simulink model "MiniDroneLogicalArchitecture"  (R2022a)
settings: Solver=VariableStepAuto  StartTime=0.0  StopTime=10.0  RelTol=1e-3
settings Model: DataDictionary=MiniDroneArchData.sldd  Creator=tshifera  LastModifiedBy=tobia

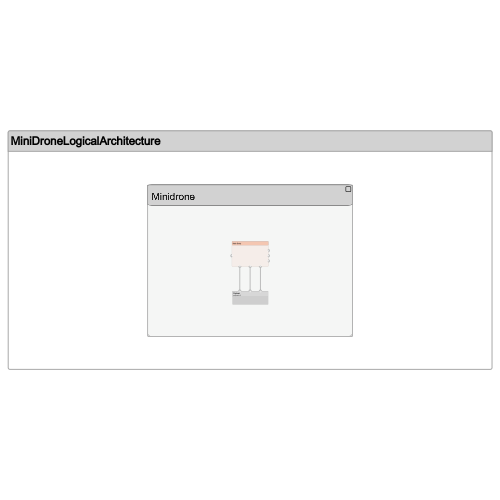
[thumbnail: Simulink's stored preview of the top-level diagram]
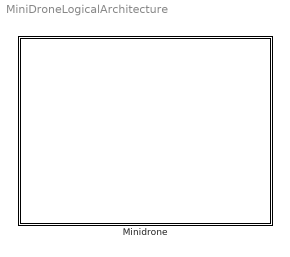
== system MiniDroneLogicalArchitecture ==
  Minidrone : Subsystem
      settings: PortSchema="{\"entries\":[{\"content\":{\"headerSize\":26,\"margin\":15,\"minimumSpacing\":25,\"sides\":[{\"content\":{\"connectorIds\":[]},\"type\":\"ConnectorPlacement.EquallySpacedRectSide\",\"uuid\":\"58971a95-43ec-4e42-90cb-f52848a43a78\"},{\"content\":{\"connectorIds\":[],\"side\":\"RIGHT\"},\"type\":\"ConnectorPlacement.EquallySpacedRectSide\",\"uuid\":\"43bd139b-3ebd-443e-9d04-2758c166e5e5\"},{\"content\":{\"connectorIds\":[],\"side\":\"TOP\"},\"type\":\"ConnectorPlacement.EquallySpacedRectSide\",\"uuid\":\"9440dd5a-d47a-4e7e-9dec-7137884490cd\"}]},\"type\":\"ConnectorPlacement.EquallySpacedConnector\",\"uuid\":\"fbcd83c6-9a27-4688-9f1d-1a4d28d86620\"}],\"packageUris\":[\"http://schema.mathworks.com/mf0/Connector/R2020b\"],\"version\":\"1.0\"}"

== system MiniDroneLogicalArchitecture/Minidrone ==
  Main Vehicle : Subsystem
      settings: PortSchema="{\"entries\":[{\"content\":{\"headerSize\":26,\"margin\":15,\"minimumSpacing\":25,\"sides\":[{\"content\":{\"connectorIds\":[\"In2\"]},\"type\":\"ConnectorPlacement.EquallySpacedRectSide\",\"uuid\":\"58971a95-43ec-4e42-90cb-f52848a43a78\"},{\"content\":{\"connectorIds\":[\"Out1\",\"Out2\",\"Out5\"],\"side\":\"RIGHT\"},\"type\":\"ConnectorPlacement.EquallySpacedRectSide\",\"uuid\":\"43bd139b-3ebd-443e-9d04-2758c166e5e5\"},{\"content\":{\"connectorIds\":[],\"side\":\"TOP\"},\"type\":\"ConnectorPlacement.EquallySpacedRectSide\",\"uuid\":\"9440dd5a-d47a-4e7e-9dec-7137884490cd\"},{\"content\":{\"connectorIds\":[\"Out3\",\"Out4\",\"In1\"],\"side\":\"BOTTOM\"},\"type\":\"ConnectorPlacement.EquallySpacedRectSide\",\"uuid\":\"027f250f-1c99-4780-b31a-0472dacd58c4\"}]},\"type\":\"ConnectorPlacement.EquallySpacedConnector\",\"uuid\":\"fbcd83c6-9a27-4688-9f1d-1a4d28d86620\"}],\"packageUris\":[\"http://schema.mathworks.com/mf0/Connector/R2020b\"],\"version\":\"1.0\"}"
  Payload : Subsystem  Variant=on
      settings: PortSchema="{\"entries\":[{\"content\":{\"headerSize\":38,\"margin\":15,\"minimumSpacing\":25,\"sides\":[{\"content\":{\"connectorIds\":[]},\"type\":\"ConnectorPlacement.EquallySpacedRectSide\",\"uuid\":\"bb20ca61-cc69-46ba-bbf8-c616735728e4\"},{\"content\":{\"connectorIds\":[],\"side\":\"RIGHT\"},\"type\":\"ConnectorPlacement.EquallySpacedRectSide\",\"uuid\":\"ae599026-5f79-458c-a34f-615f09cd605e\"},{\"content\":{\"connectorIds\":[\"In1\",\"In2\",\"Out1\"],\"side\":\"TOP\"},\"type\":\"ConnectorPlacement.EquallySpacedRectSide\",\"uuid\":\"37784589-cb93-414b-b17d-4791bb265658\"}]},\"type\":\"ConnectorPlacement.EquallySpacedConnector\",\"uuid\":\"a9e16083-13fe-49b9-9fa3-3eed0fc58f12\"}],\"packageUris\":[\"http://schema.mathworks.com/mf0/Connector/R2020b\"],\"version\":\"1.0\"}"
  wires:
  Main Vehicle/3(PL Coupling) -> Payload/1(PL Coupling)
  Main Vehicle/4(PL Command) -> Payload/2(PL Command)
  Payload/1(PL State) -> Main Vehicle/1(PL State)

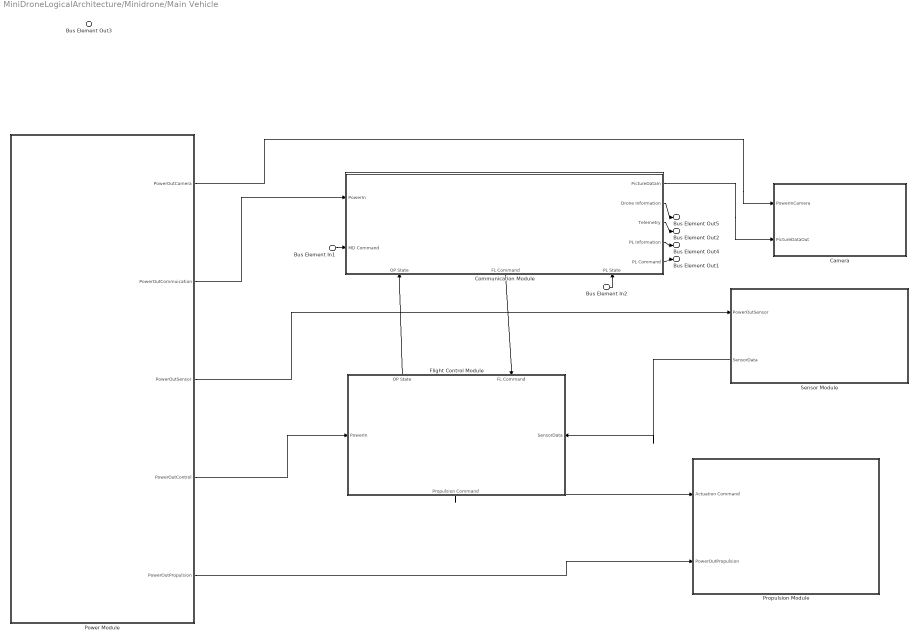
== system MiniDroneLogicalArchitecture/Minidrone/Main Vehicle ==
  Bus Element In2 : Inport  PortName=PL State
  Bus Element In1 : Inport  Port=2  PortName=MD Command
  Camera : Subsystem  VariantControl=payload==1
      settings: PortSchema="{\"entries\":[{\"content\":{\"headerSize\":26,\"margin\":15,\"minimumSpacing\":25,\"sides\":[{\"content\":{\"connectorIds\":[\"In1\",\"In2\"]},\"type\":\"ConnectorPlacement.EquallySpacedRectSide\",\"uuid\":\"62dbea54-6b04-428b-9082-afe16aec4c16\"},{\"content\":{\"connectorIds\":[],\"side\":\"RIGHT\"},\"type\":\"ConnectorPlacement.EquallySpacedRectSide\",\"uuid\":\"bd8afa16-d094-436c-bc9f-80902768e85a\"},{\"content\":{\"connectorIds\":[],\"side\":\"TOP\"},\"type\":\"ConnectorPlacement.EquallySpacedRectSide\",\"uuid\":\"5bc22b2d-7b46-48f6-9c81-aea78f4cffe8\"}]},\"type\":\"ConnectorPlacement.EquallySpacedConnector\",\"uuid\":\"869dc23c-b8e9-4489-a84c-3bf9ddec322d\"}],\"packageUris\":[\"http://schema.mathworks.com/mf0/Connector/R2020b\"],\"version\":\"1.0\"}"
  Communication Module : Subsystem
      settings: PortSchema="{\"entries\":[{\"content\":{\"headerSize\":26,\"margin\":15,\"minimumSpacing\":25,\"sides\":[{\"content\":{\"connectorIds\":[\"In3\",\"In4\"]},\"type\":\"ConnectorPlacement.EquallySpacedRectSide\",\"uuid\":\"11745183-c785-42ff-bcc1-ca3285cfe892\"},{\"content\":{\"connectorIds\":[\"Out1\",\"Out2\",\"Out6\",\"Out4\",\"Out5\"],\"side\":\"RIGHT\"},\"type\":\"ConnectorPlacement.EquallySpacedRectSide\",\"uuid\":\"762d8cad-319e-4e1e-8739-8b76a70aa4c0\"},{\"content\":{\"connectorIds\":[],\"side\":\"TOP\"},\"type\":\"ConnectorPlacement.EquallySpacedRectSide\",\"uuid\":\"cf327f13-56fb-47e7-82e2-9b80047871fd\"},{\"content\":{\"connectorIds\":[\"In1\",\"Out3\",\"In2\"],\"side\":\"BOTTOM\"},\"type\":\"ConnectorPlacement.EquallySpacedRectSide\",\"uuid\":\"b154881a-f2db-4811-b63b-30ed04e21acf\"}]},\"type\":\"ConnectorPlacement.EquallySpacedConnector\",\"uuid\":\"6e856333-11ed-42a7-b683-e6a750f8e1be\"}],\"packageUris\":[\"http://schema.mathworks.com/mf0/Connector/R2020b\"],\"version\":\"1.0\"}"
  Flight Control Module : Subsystem
      settings: PortSchema="{\"entries\":[{\"content\":{\"headerSize\":26,\"margin\":15,\"minimumSpacing\":25,\"sides\":[{\"content\":{\"connectorIds\":[\"In2\"]},\"type\":\"ConnectorPlacement.EquallySpacedRectSide\",\"uuid\":\"11745183-c785-42ff-bcc1-ca3285cfe892\"},{\"content\":{\"connectorIds\":[\"In3\"],\"side\":\"RIGHT\"},\"type\":\"ConnectorPlacement.EquallySpacedRectSide\",\"uuid\":\"762d8cad-319e-4e1e-8739-8b76a70aa4c0\"},{\"content\":{\"connectorIds\":[\"Out1\",\"In1\"],\"side\":\"TOP\"},\"type\":\"ConnectorPlacement.EquallySpacedRectSide\",\"uuid\":\"cf327f13-56fb-47e7-82e2-9b80047871fd\"},{\"content\":{\"connectorIds\":[\"Out2\"],\"side\":\"BOTTOM\"},\"type\":\"ConnectorPlacement.EquallySpacedRectSide\",\"uuid\":\"d4b2c298-dd23-4e2a-8fa6-8732704f5c39\"}]},\"type\":\"ConnectorPlacement.EquallySpacedConnector\",\"uuid\":\"6e856333-11ed-42a7-b683-e6a750f8e1be\"}],\"packageUris\":[\"http://schema.mathworks.com/mf0/Connector/R2020b\"],\"version\":\"1.0\"}"
  Power Module : Subsystem
      settings: PortSchema="{\"entries\":[{\"content\":{\"headerSize\":26,\"margin\":15,\"minimumSpacing\":25,\"sides\":[{\"content\":{\"connectorIds\":[]},\"type\":\"ConnectorPlacement.EquallySpacedRectSide\",\"uuid\":\"11745183-c785-42ff-bcc1-ca3285cfe892\"},{\"content\":{\"connectorIds\":[\"Out1\",\"Out5\",\"Out3\",\"Out2\",\"Out4\"],\"side\":\"RIGHT\"},\"type\":\"ConnectorPlacement.EquallySpacedRectSide\",\"uuid\":\"762d8cad-319e-4e1e-8739-8b76a70aa4c0\"},{\"content\":{\"connectorIds\":[],\"side\":\"TOP\"},\"type\":\"ConnectorPlacement.EquallySpacedRectSide\",\"uuid\":\"cf327f13-56fb-47e7-82e2-9b80047871fd\"}]},\"type\":\"ConnectorPlacement.EquallySpacedConnector\",\"uuid\":\"6e856333-11ed-42a7-b683-e6a750f8e1be\"}],\"packageUris\":[\"http://schema.mathworks.com/mf0/Connector/R2020b\"],\"version\":\"1.0\"}"
  Propulsion Module : Subsystem
      settings: PortSchema="{\"entries\":[{\"content\":{\"headerSize\":26,\"margin\":15,\"minimumSpacing\":25,\"sides\":[{\"content\":{\"connectorIds\":[\"In1\",\"In2\"]},\"type\":\"ConnectorPlacement.EquallySpacedRectSide\",\"uuid\":\"11745183-c785-42ff-bcc1-ca3285cfe892\"},{\"content\":{\"connectorIds\":[],\"side\":\"RIGHT\"},\"type\":\"ConnectorPlacement.EquallySpacedRectSide\",\"uuid\":\"762d8cad-319e-4e1e-8739-8b76a70aa4c0\"},{\"content\":{\"connectorIds\":[],\"side\":\"TOP\"},\"type\":\"ConnectorPlacement.EquallySpacedRectSide\",\"uuid\":\"cf327f13-56fb-47e7-82e2-9b80047871fd\"}]},\"type\":\"ConnectorPlacement.EquallySpacedConnector\",\"uuid\":\"6e856333-11ed-42a7-b683-e6a750f8e1be\"}],\"packageUris\":[\"http://schema.mathworks.com/mf0/Connector/R2020b\"],\"version\":\"1.0\"}"
  Sensor Module : Subsystem
      settings: PortSchema="{\"entries\":[{\"content\":{\"headerSize\":26,\"margin\":15,\"minimumSpacing\":25,\"sides\":[{\"content\":{\"connectorIds\":[\"In1\",\"Out1\"]},\"type\":\"ConnectorPlacement.EquallySpacedRectSide\",\"uuid\":\"11745183-c785-42ff-bcc1-ca3285cfe892\"},{\"content\":{\"connectorIds\":[],\"side\":\"RIGHT\"},\"type\":\"ConnectorPlacement.EquallySpacedRectSide\",\"uuid\":\"762d8cad-319e-4e1e-8739-8b76a70aa4c0\"},{\"content\":{\"connectorIds\":[],\"side\":\"TOP\"},\"type\":\"ConnectorPlacement.EquallySpacedRectSide\",\"uuid\":\"cf327f13-56fb-47e7-82e2-9b80047871fd\"}]},\"type\":\"ConnectorPlacement.EquallySpacedConnector\",\"uuid\":\"6e856333-11ed-42a7-b683-e6a750f8e1be\"}],\"packageUris\":[\"http://schema.mathworks.com/mf0/Connector/R2020b\"],\"version\":\"1.0\"}"
  Bus Element Out5 : Outport  PortName=Drone Information
  Bus Element Out4 : Outport  Port=2  PortName=PL Information
  Bus Element Out3 : Outport  Port=3  PortName=PL Coupling
  Bus Element Out1 : Outport  Port=4  PortName=PL Command
  Bus Element Out2 : Outport  Port=5  PortName=Telemetry
  wires:
  Bus Element In1/1 -> Communication Module/4(MD Command)
  Communication Module/3(FL Command) -> Flight Control Module/1(FL Command)
  Power Module/5(PowerOutCommuication) -> Communication Module/3(PowerIn)
  Power Module/2(PowerOutControl) -> Flight Control Module/2(PowerIn)
  Power Module/4(PowerOutPropulsion) -> Propulsion Module/2(PowerOutPropulsion)
  Communication Module/6(Telemetry) -> Bus Element Out2/1
  Flight Control Module/1(OP State) -> Communication Module/1(OP State)
  Communication Module/5(PL Command) -> Bus Element Out1/1
  Bus Element In2/1 -> Communication Module/2(PL State)
  Communication Module/4(PL Information) -> Bus Element Out4/1
  Communication Module/2(Drone Information) -> Bus Element Out5/1
  Sensor Module/1(SensorData) -> Flight Control Module/3(SensorData)
  Flight Control Module/2(Propulsion Command) -> Propulsion Module/1(Actuation Command)
  Power Module/3(PowerOutSensor) -> Sensor Module/1(PowerOutSensor)
  Power Module/1(PowerOutCamera) -> Camera/1(PowerInCamera)
  Communication Module/1(PictureDataIn) -> Camera/2(PictureDataOut)

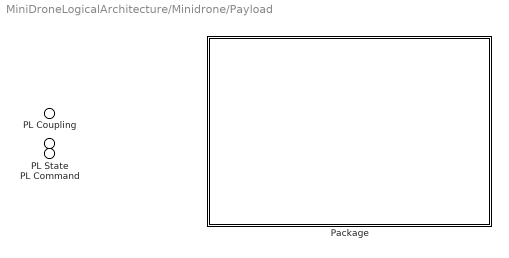
== system MiniDroneLogicalArchitecture/Minidrone/Payload ==
  PL Coupling : Inport
  PL Command : Inport  Port=2
  Package : Subsystem  VariantControl=payload==2
      settings: PortSchema="{\"entries\":[{\"content\":{\"headerSize\":26,\"margin\":15,\"minimumSpacing\":25,\"sides\":[{\"content\":{\"connectorIds\":[]},\"type\":\"ConnectorPlacement.EquallySpacedRectSide\",\"uuid\":\"62dbea54-6b04-428b-9082-afe16aec4c16\"},{\"content\":{\"connectorIds\":[],\"side\":\"RIGHT\"},\"type\":\"ConnectorPlacement.EquallySpacedRectSide\",\"uuid\":\"bd8afa16-d094-436c-bc9f-80902768e85a\"},{\"content\":{\"connectorIds\":[],\"side\":\"TOP\"},\"type\":\"ConnectorPlacement.EquallySpacedRectSide\",\"uuid\":\"5bc22b2d-7b46-48f6-9c81-aea78f4cffe8\"}]},\"type\":\"ConnectorPlacement.EquallySpacedConnector\",\"uuid\":\"869dc23c-b8e9-4489-a84c-3bf9ddec322d\"}],\"packageUris\":[\"http://schema.mathworks.com/mf0/Connector/R2020b\"],\"version\":\"1.0\"}"
  PL State : Outport

== system MiniDroneLogicalArchitecture/Minidrone/Main Vehicle/Camera ==
  Bus Element In1 : Inport  PortName=PowerInCamera
  Bus Element In2 : Inport  Port=2  PortName=PictureDataOut

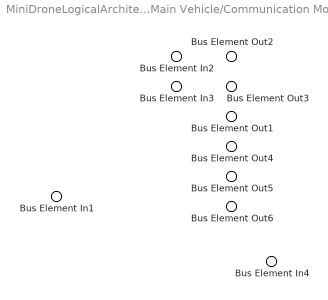
== system MiniDroneLogicalArchitecture/Minidrone/Main Vehicle/Communication Module ==
  Bus Element In4 : Inport  PortName=OP State
  Bus Element In3 : Inport  Port=2  PortName=PL State
  Bus Element In2 : Inport  Port=3  PortName=PowerIn
  Bus Element In1 : Inport  Port=4  PortName=MD Command
  Bus Element Out6 : Outport  PortName=PictureDataIn
  Bus Element Out5 : Outport  Port=2  PortName=Drone Information
  Bus Element Out2 : Outport  Port=3  PortName=FL Command
  Bus Element Out4 : Outport  Port=4  PortName=PL Information
  Bus Element Out1 : Outport  Port=5  PortName=PL Command
  Bus Element Out3 : Outport  Port=6  PortName=Telemetry

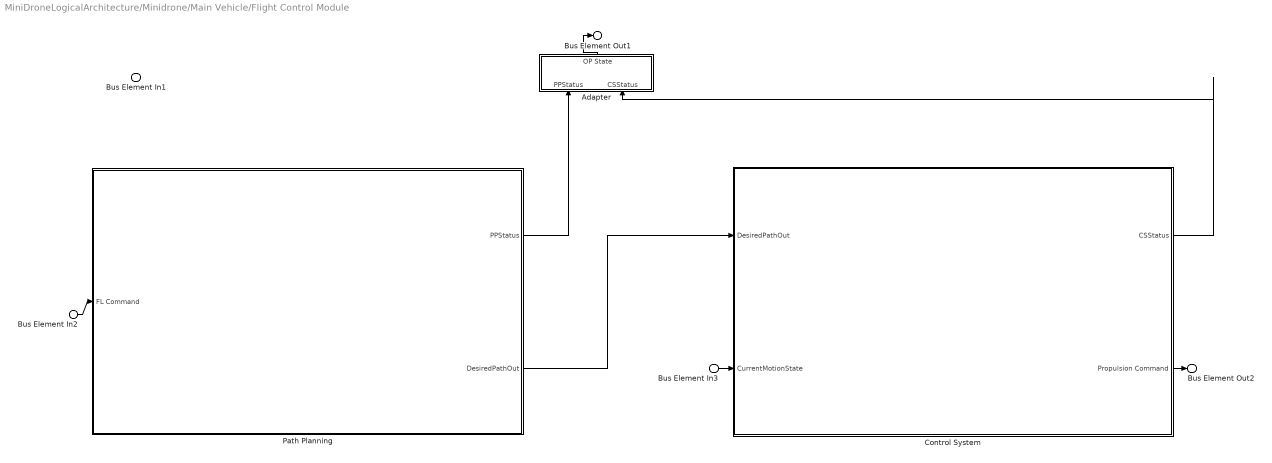
== system MiniDroneLogicalArchitecture/Minidrone/Main Vehicle/Flight Control Module ==
  Bus Element In2 : Inport  PortName=FL Command
  Bus Element In1 : Inport  Port=2  PortName=PowerIn
  Bus Element In3 : Inport  Port=3  PortName=SensorData
  Adapter : Subsystem
      settings: PortSchema="{\"entries\":[{\"content\":{\"margin\":10,\"minimumSpacing\":15,\"sides\":[{\"content\":{\"connectorIds\":[]},\"type\":\"ConnectorPlacement.EquallySpacedRectSide\",\"uuid\":\"8029eac4-1e93-42cb-93bf-2741aac18114\"},{\"content\":{\"connectorIds\":[],\"side\":\"RIGHT\"},\"type\":\"ConnectorPlacement.EquallySpacedRectSide\",\"uuid\":\"880550d5-d396-4c9d-9596-cf9ff815056e\"},{\"content\":{\"connectorIds\":[\"Out1\"],\"side\":\"TOP\"},\"type\":\"ConnectorPlacement.EquallySpacedRectSide\",\"uuid\":\"ddd57148-5a11-4830-bb53-0e7c5eb0188d\"},{\"content\":{\"connectorIds\":[\"In1\",\"In2\"],\"side\":\"BOTTOM\"},\"type\":\"ConnectorPlacement.EquallySpacedRectSide\",\"uuid\":\"686e057f-801d-4689-adbf-8d23a9ad6c3b\"}]},\"type\":\"ConnectorPlacement.EquallySpacedConnector\",\"uuid\":\"9cd7aed1-ed17-433b-a42b-f5bc10fbd0dd\"}],\"packageUris\":[\"http://schema.mathworks.com/mf0/Connector/R2020b\"],\"version\":\"1.0\"}"
  Control System : Subsystem
      settings: PortSchema="{\"entries\":[{\"content\":{\"headerSize\":26,\"margin\":15,\"minimumSpacing\":25,\"sides\":[{\"content\":{\"connectorIds\":[\"In1\",\"In2\"]},\"type\":\"ConnectorPlacement.EquallySpacedRectSide\",\"uuid\":\"11745183-c785-42ff-bcc1-ca3285cfe892\"},{\"content\":{\"connectorIds\":[\"Out1\",\"Out2\"],\"side\":\"RIGHT\"},\"type\":\"ConnectorPlacement.EquallySpacedRectSide\",\"uuid\":\"762d8cad-319e-4e1e-8739-8b76a70aa4c0\"},{\"content\":{\"connectorIds\":[],\"side\":\"TOP\"},\"type\":\"ConnectorPlacement.EquallySpacedRectSide\",\"uuid\":\"cf327f13-56fb-47e7-82e2-9b80047871fd\"}]},\"type\":\"ConnectorPlacement.EquallySpacedConnector\",\"uuid\":\"6e856333-11ed-42a7-b683-e6a750f8e1be\"}],\"packageUris\":[\"http://schema.mathworks.com/mf0/Connector/R2020b\"],\"version\":\"1.0\"}"
  Path Planning : Subsystem
      settings: PortSchema="{\"entries\":[{\"content\":{\"headerSize\":26,\"margin\":15,\"minimumSpacing\":25,\"sides\":[{\"content\":{\"connectorIds\":[\"In1\"]},\"type\":\"ConnectorPlacement.EquallySpacedRectSide\",\"uuid\":\"11745183-c785-42ff-bcc1-ca3285cfe892\"},{\"content\":{\"connectorIds\":[\"Out1\",\"Out2\"],\"side\":\"RIGHT\"},\"type\":\"ConnectorPlacement.EquallySpacedRectSide\",\"uuid\":\"762d8cad-319e-4e1e-8739-8b76a70aa4c0\"},{\"content\":{\"connectorIds\":[],\"side\":\"TOP\"},\"type\":\"ConnectorPlacement.EquallySpacedRectSide\",\"uuid\":\"cf327f13-56fb-47e7-82e2-9b80047871fd\"}]},\"type\":\"ConnectorPlacement.EquallySpacedConnector\",\"uuid\":\"6e856333-11ed-42a7-b683-e6a750f8e1be\"}],\"packageUris\":[\"http://schema.mathworks.com/mf0/Connector/R2020b\"],\"version\":\"1.0\"}"
  Bus Element Out1 : Outport  PortName=OP State
  Bus Element Out2 : Outport  Port=2  PortName=Propulsion Command
  wires:
  Bus Element In2/1 -> Path Planning/1(FL Command)
  Path Planning/2(DesiredPathOut) -> Control System/1(DesiredPathOut)
  Bus Element In3/1 -> Control System/2(CurrentMotionState)
  Control System/2(Propulsion Command) -> Bus Element Out2/1
  Adapter/1(OP State) -> Bus Element Out1/1
  Path Planning/1(PPStatus) -> Adapter/1(PPStatus)
  Control System/1(CSStatus) -> Adapter/2(CSStatus)

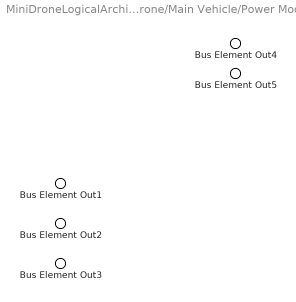
== system MiniDroneLogicalArchitecture/Minidrone/Main Vehicle/Power Module ==
  Bus Element Out5 : Outport  PortName=PowerOutCamera
  Bus Element Out1 : Outport  Port=2  PortName=PowerOutControl
  Bus Element Out4 : Outport  Port=3  PortName=PowerOutSensor
  Bus Element Out2 : Outport  Port=4  PortName=PowerOutPropulsion
  Bus Element Out3 : Outport  Port=5  PortName=PowerOutCommuication

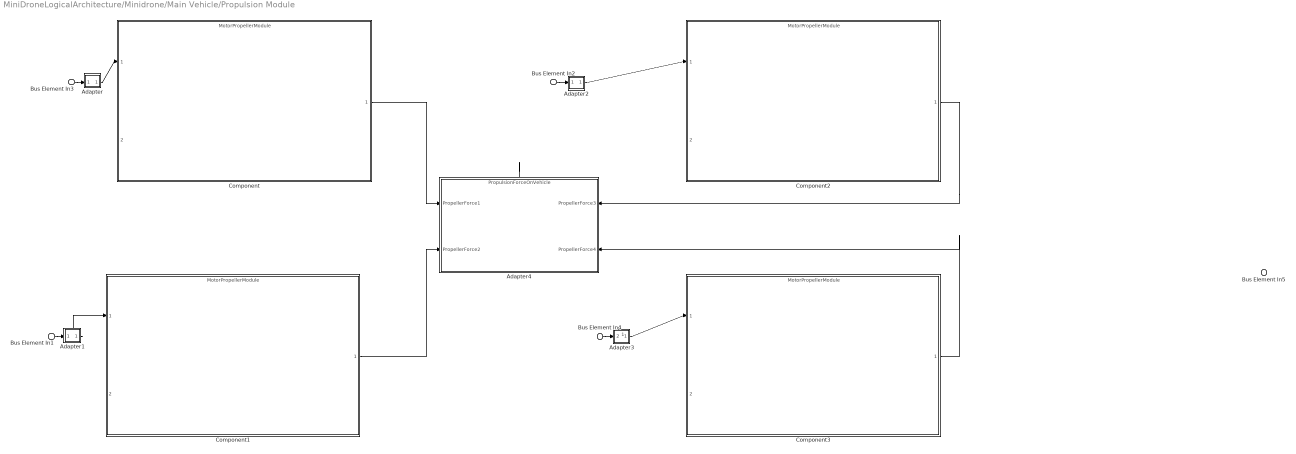
== system MiniDroneLogicalArchitecture/Minidrone/Main Vehicle/Propulsion Module ==
  Bus Element In{1..4} (4 alike) : Inport  PortName=Actuation Command
  Bus Element In5 : Inport  Port=2  PortName=PowerOutPropulsion
  Adapter : Subsystem
      settings: PortSchema="{\"entries\":[{\"content\":{\"margin\":10,\"minimumSpacing\":15,\"sides\":[{\"content\":{\"connectorIds\":[\"In1\"]},\"type\":\"ConnectorPlacement.EquallySpacedRectSide\",\"uuid\":\"8029eac4-1e93-42cb-93bf-2741aac18114\"},{\"content\":{\"connectorIds\":[\"Out1\"],\"side\":\"RIGHT\"},\"type\":\"ConnectorPlacement.EquallySpacedRectSide\",\"uuid\":\"880550d5-d396-4c9d-9596-cf9ff815056e\"},{\"content\":{\"connectorIds\":[],\"side\":\"TOP\"},\"type\":\"ConnectorPlacement.EquallySpacedRectSide\",\"uuid\":\"ddd57148-5a11-4830-bb53-0e7c5eb0188d\"}]},\"type\":\"ConnectorPlacement.EquallySpacedConnector\",\"uuid\":\"9cd7aed1-ed17-433b-a42b-f5bc10fbd0dd\"}],\"packageUris\":[\"http://schema.mathworks.com/mf0/Connector/R2020b\"],\"version\":\"1.0\"}"
  Adapter1 : Subsystem
      settings: PortSchema="{\"entries\":[{\"content\":{\"margin\":10,\"minimumSpacing\":15,\"sides\":[{\"content\":{\"connectorIds\":[\"In1\"]},\"type\":\"ConnectorPlacement.EquallySpacedRectSide\",\"uuid\":\"8029eac4-1e93-42cb-93bf-2741aac18114\"},{\"content\":{\"connectorIds\":[\"Out1\"],\"side\":\"RIGHT\"},\"type\":\"ConnectorPlacement.EquallySpacedRectSide\",\"uuid\":\"880550d5-d396-4c9d-9596-cf9ff815056e\"},{\"content\":{\"connectorIds\":[],\"side\":\"TOP\"},\"type\":\"ConnectorPlacement.EquallySpacedRectSide\",\"uuid\":\"ddd57148-5a11-4830-bb53-0e7c5eb0188d\"}]},\"type\":\"ConnectorPlacement.EquallySpacedConnector\",\"uuid\":\"9cd7aed1-ed17-433b-a42b-f5bc10fbd0dd\"}],\"packageUris\":[\"http://schema.mathworks.com/mf0/Connector/R2020b\"],\"version\":\"1.0\"}"
  Adapter2 : Subsystem
      settings: PortSchema="{\"entries\":[{\"content\":{\"margin\":10,\"minimumSpacing\":15,\"sides\":[{\"content\":{\"connectorIds\":[\"In1\"]},\"type\":\"ConnectorPlacement.EquallySpacedRectSide\",\"uuid\":\"8029eac4-1e93-42cb-93bf-2741aac18114\"},{\"content\":{\"connectorIds\":[\"Out1\"],\"side\":\"RIGHT\"},\"type\":\"ConnectorPlacement.EquallySpacedRectSide\",\"uuid\":\"880550d5-d396-4c9d-9596-cf9ff815056e\"},{\"content\":{\"connectorIds\":[],\"side\":\"TOP\"},\"type\":\"ConnectorPlacement.EquallySpacedRectSide\",\"uuid\":\"ddd57148-5a11-4830-bb53-0e7c5eb0188d\"}]},\"type\":\"ConnectorPlacement.EquallySpacedConnector\",\"uuid\":\"9cd7aed1-ed17-433b-a42b-f5bc10fbd0dd\"}],\"packageUris\":[\"http://schema.mathworks.com/mf0/Connector/R2020b\"],\"version\":\"1.0\"}"
  Adapter3 : Subsystem
      settings: PortSchema="{\"entries\":[{\"content\":{\"margin\":10,\"minimumSpacing\":15,\"sides\":[{\"content\":{\"connectorIds\":[\"In2\"]},\"type\":\"ConnectorPlacement.EquallySpacedRectSide\",\"uuid\":\"8029eac4-1e93-42cb-93bf-2741aac18114\"},{\"content\":{\"connectorIds\":[\"Out1\"],\"side\":\"RIGHT\"},\"type\":\"ConnectorPlacement.EquallySpacedRectSide\",\"uuid\":\"880550d5-d396-4c9d-9596-cf9ff815056e\"},{\"content\":{\"connectorIds\":[\"In1\"],\"side\":\"TOP\"},\"type\":\"ConnectorPlacement.EquallySpacedRectSide\",\"uuid\":\"ddd57148-5a11-4830-bb53-0e7c5eb0188d\"}]},\"type\":\"ConnectorPlacement.EquallySpacedConnector\",\"uuid\":\"9cd7aed1-ed17-433b-a42b-f5bc10fbd0dd\"}],\"packageUris\":[\"http://schema.mathworks.com/mf0/Connector/R2020b\"],\"version\":\"1.0\"}"
  Adapter4 : Subsystem
      settings: PortSchema="{\"entries\":[{\"content\":{\"margin\":10,\"minimumSpacing\":15,\"sides\":[{\"content\":{\"connectorIds\":[\"In4\",\"In3\"]},\"type\":\"ConnectorPlacement.EquallySpacedRectSide\",\"uuid\":\"b95fdf5c-7c32-4cea-a1d5-46e14885b6c7\"},{\"content\":{\"connectorIds\":[\"In1\",\"In2\"],\"side\":\"RIGHT\"},\"type\":\"ConnectorPlacement.EquallySpacedRectSide\",\"uuid\":\"406c0812-4108-47cf-89cd-ae4270ca37a8\"},{\"content\":{\"connectorIds\":[\"Out1\"],\"side\":\"TOP\"},\"type\":\"ConnectorPlacement.EquallySpacedRectSide\",\"uuid\":\"1ebf6b83-00c0-4ac6-93de-25d0ef6ef9e5\"}]},\"type\":\"ConnectorPlacement.EquallySpacedConnector\",\"uuid\":\"7218703e-d378-431b-88e9-2d6710b1e02c\"}],\"packageUris\":[\"http://schema.mathworks.com/mf0/Connector/R2020b\"],\"version\":\"1.0\"}"
  Component{,1..3} (4 alike) : ModelReference  ModelNameDialog=MotorPropellerModule.slx  SimulationMode=Normal  ModelReferenceVersion=1.7
      settings: PortSchema="{\"entries\":[{\"content\":{\"headerSize\":38,\"margin\":15,\"minimumSpacing\":25,\"sides\":[{\"content\":{\"connectorIds\":[\"In1\",\"In2\"]},\"type\":\"ConnectorPlacement.EquallySpacedRectSide\",\"uuid\":\"7b7af72e-aa04-46fd-a07e-d8d59d662379\"},{\"content\":{\"connectorIds\":[\"Out1\"],\"side\":\"RIGHT\"},\"type\":\"ConnectorPlacement.EquallySpacedRectSide\",\"uuid\":\"fdfbdd79-f6fe-4609-8655-22f9d8d17dc0\"},{\"content\":{\"connectorIds\":[],\"side\":\"TOP\"},\"type\":\"ConnectorPlacement.EquallySpacedRectSide\",\"uuid\":\"626fe178-dafd-47c5-aa64-f4cd4b451539\"}]},\"type\":\"ConnectorPlacement.EquallySpacedConnector\",\"uuid\":\"b35cf388-f6ba-41d8-a395-5e8a060747f6\"}],\"packageUris\":[\"http://schema.mathworks.com/mf0/Connector/R2020b\"],\"version\":\"1.0\"}"
  wires:
  Adapter/1(MotorCommand) -> Component/1
  Bus Element In3/1 -> Adapter/1(Actuation Command)
  Adapter1/1(MotorCommand) -> Component1/1
  Bus Element In1/1 -> Adapter1/1(Actuation Command)
  Adapter2/1(MotorCommand) -> Component2/1
  Bus Element In2/1 -> Adapter2/1(Actuation Command)
  Bus Element In4/1 -> Adapter3/2(Actuation Command)
  Adapter3/1(MotorCommand) -> Component3/1
  Adapter4/1(PropulsionForceOnVehicle) -> ?
  Component2/1 -> Adapter4/1(PropellerForce3)
  Component3/1 -> Adapter4/2(PropellerForce4)
  Component1/1 -> Adapter4/3(PropellerForce2)
  Component/1 -> Adapter4/4(PropellerForce1)

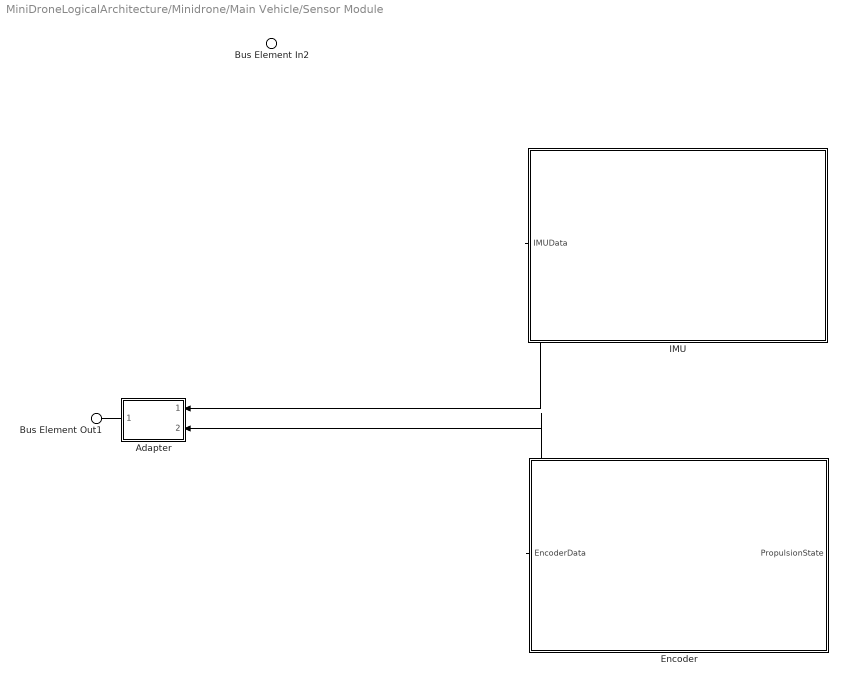
== system MiniDroneLogicalArchitecture/Minidrone/Main Vehicle/Sensor Module ==
  Bus Element In2 : Inport  PortName=PowerOutSensor
  Adapter : Subsystem
      settings: PortSchema="{\"entries\":[{\"content\":{\"margin\":10,\"minimumSpacing\":15,\"sides\":[{\"content\":{\"connectorIds\":[\"Out1\"]},\"type\":\"ConnectorPlacement.EquallySpacedRectSide\",\"uuid\":\"58971a95-43ec-4e42-90cb-f52848a43a78\"},{\"content\":{\"connectorIds\":[\"In1\",\"In2\"],\"side\":\"RIGHT\"},\"type\":\"ConnectorPlacement.EquallySpacedRectSide\",\"uuid\":\"43bd139b-3ebd-443e-9d04-2758c166e5e5\"},{\"content\":{\"connectorIds\":[],\"side\":\"TOP\"},\"type\":\"ConnectorPlacement.EquallySpacedRectSide\",\"uuid\":\"9440dd5a-d47a-4e7e-9dec-7137884490cd\"},{\"content\":{\"connectorIds\":[],\"side\":\"BOTTOM\"},\"type\":\"ConnectorPlacement.EquallySpacedRectSide\",\"uuid\":\"a500e90f-9d10-4320-8532-1d80de54d601\"}]},\"type\":\"ConnectorPlacement.EquallySpacedConnector\",\"uuid\":\"fbcd83c6-9a27-4688-9f1d-1a4d28d86620\"}],\"packageUris\":[\"http://schema.mathworks.com/mf0/Connector/R2020b\"],\"version\":\"1.0\"}"
  Encoder : Subsystem
      settings: PortSchema="{\"entries\":[{\"content\":{\"headerSize\":26,\"margin\":15,\"minimumSpacing\":25,\"sides\":[{\"content\":{\"connectorIds\":[\"Out1\"]},\"type\":\"ConnectorPlacement.EquallySpacedRectSide\",\"uuid\":\"58971a95-43ec-4e42-90cb-f52848a43a78\"},{\"content\":{\"connectorIds\":[\"In1\"],\"side\":\"RIGHT\"},\"type\":\"ConnectorPlacement.EquallySpacedRectSide\",\"uuid\":\"43bd139b-3ebd-443e-9d04-2758c166e5e5\"},{\"content\":{\"connectorIds\":[],\"side\":\"TOP\"},\"type\":\"ConnectorPlacement.EquallySpacedRectSide\",\"uuid\":\"9440dd5a-d47a-4e7e-9dec-7137884490cd\"}]},\"type\":\"ConnectorPlacement.EquallySpacedConnector\",\"uuid\":\"fbcd83c6-9a27-4688-9f1d-1a4d28d86620\"}],\"packageUris\":[\"http://schema.mathworks.com/mf0/Connector/R2020b\"],\"version\":\"1.0\"}"
  "IMU " : Subsystem
      settings: PortSchema="{\"entries\":[{\"content\":{\"headerSize\":26,\"margin\":15,\"minimumSpacing\":25,\"sides\":[{\"content\":{\"connectorIds\":[\"Out1\"]},\"type\":\"ConnectorPlacement.EquallySpacedRectSide\",\"uuid\":\"58971a95-43ec-4e42-90cb-f52848a43a78\"},{\"content\":{\"connectorIds\":[],\"side\":\"RIGHT\"},\"type\":\"ConnectorPlacement.EquallySpacedRectSide\",\"uuid\":\"43bd139b-3ebd-443e-9d04-2758c166e5e5\"},{\"content\":{\"connectorIds\":[],\"side\":\"TOP\"},\"type\":\"ConnectorPlacement.EquallySpacedRectSide\",\"uuid\":\"9440dd5a-d47a-4e7e-9dec-7137884490cd\"}]},\"type\":\"ConnectorPlacement.EquallySpacedConnector\",\"uuid\":\"fbcd83c6-9a27-4688-9f1d-1a4d28d86620\"}],\"packageUris\":[\"http://schema.mathworks.com/mf0/Connector/R2020b\"],\"version\":\"1.0\"}"
  Bus Element Out1 : Outport  PortName=SensorData
  wires:
  ? -> Encoder/1(PropulsionState)
  Adapter/1(SensorData) -> Bus Element Out1/1
  "IMU "/1(IMUData) -> Adapter/1(IMUData)
  Encoder/1(EncoderData) -> Adapter/2(EncoderData)

== system MiniDroneLogicalArchitecture/Minidrone/Payload/Package ==

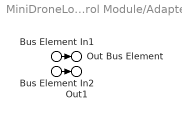
== system MiniDroneLogicalArchitecture/Minidrone/Main Vehicle/Flight Control Module/Adapter ==
  Bus Element In1 : Inport  PortName=PPStatus
  Bus Element In2 : Inport  Port=2  PortName=CSStatus
  Out Bus Element : Outport  PortName=OP State  Element=PPStatus
  Out1 : Outport  PortName=OP State  Element=CSStatus
  wires:
  Bus Element In1/1 -> Out Bus Element/1
  Bus Element In2/1 -> Out1/1

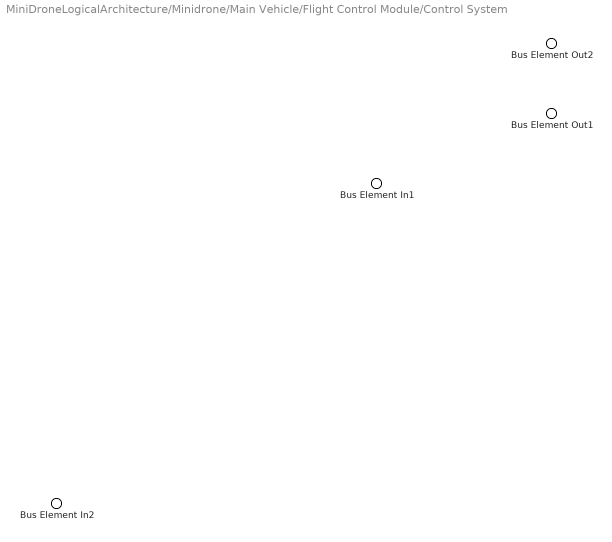
== system MiniDroneLogicalArchitecture/Minidrone/Main Vehicle/Flight Control Module/Control System ==
  Bus Element In1 : Inport  PortName=DesiredPathOut
  Bus Element In2 : Inport  Port=2  PortName=CurrentMotionState
  Bus Element Out2 : Outport  PortName=CSStatus
  Bus Element Out1 : Outport  Port=2  PortName=Propulsion Command

== system MiniDroneLogicalArchitecture/Minidrone/Main Vehicle/Flight Control Module/Path Planning ==
  Bus Element In1 : Inport  PortName=FL Command
  Bus Element Out2 : Outport  PortName=PPStatus
  Bus Element Out1 : Outport  Port=2  PortName=DesiredPathOut

== system MiniDroneLogicalArchitecture/Minidrone/Main Vehicle/Propulsion Module/Adapter ==
  In Bus Element : Inport  PortName=Actuation Command  Element=elem0
  Out Bus Element : Outport  PortName=MotorCommand
  wires:
  In Bus Element/1 -> Out Bus Element/1

== system MiniDroneLogicalArchitecture/Minidrone/Main Vehicle/Propulsion Module/Adapter1 ==
  In Bus Element : Inport  PortName=Actuation Command  Element=elem1
  Out Bus Element : Outport  PortName=MotorCommand
  wires:
  In Bus Element/1 -> Out Bus Element/1

== system MiniDroneLogicalArchitecture/Minidrone/Main Vehicle/Propulsion Module/Adapter2 ==
  In Bus Element : Inport  PortName=Actuation Command  Element=elem2
  Out Bus Element : Outport  PortName=MotorCommand
  wires:
  In Bus Element/1 -> Out Bus Element/1

== system MiniDroneLogicalArchitecture/Minidrone/Main Vehicle/Propulsion Module/Adapter3 ==
  Bus Element In1 : Inport  PortName=InBus
  In Bus Element : Inport  Port=2  PortName=Actuation Command  Element=elem3
  Out Bus Element : Outport  PortName=MotorCommand
  wires:
  In Bus Element/1 -> Out Bus Element/1

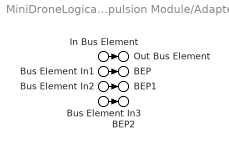
== system MiniDroneLogicalArchitecture/Minidrone/Main Vehicle/Propulsion Module/Adapter4 ==
  Bus Element In2 : Inport  PortName=PropellerForce3
  Bus Element In3 : Inport  Port=2  PortName=PropellerForce4
  Bus Element In1 : Inport  Port=3  PortName=PropellerForce2
  In Bus Element : Inport  Port=4  PortName=PropellerForce1
  Out Bus Element : Outport  PortName=PropulsionForceOnVehicle  Element=ForcePropeller1
  BEP : Outport  PortName=PropulsionForceOnVehicle  Element=ForcePropeller2
  BEP1 : Outport  PortName=PropulsionForceOnVehicle  Element=ForcePropeller3
  BEP2 : Outport  PortName=PropulsionForceOnVehicle  Element=ForcePropeller4
  wires:
  In Bus Element/1 -> Out Bus Element/1
  Bus Element In1/1 -> BEP/1
  Bus Element In2/1 -> BEP1/1
  Bus Element In3/1 -> BEP2/1

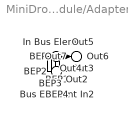
== system MiniDroneLogicalArchitecture/Minidrone/Main Vehicle/Sensor Module/Adapter ==
  In Bus Element : Inport  PortName=IMUData  Element=Acceleration
  BEP : Inport  PortName=IMUData  Element=AngularAcceleration
  BEP1 : Inport  PortName=IMUData  Element=Pose
  Bus Element In2 : Inport  Port=2  PortName=EncoderData  Element=Motor1Velocity
  BEP2 : Inport  Port=2  PortName=EncoderData  Element=Motor2Velocity
  BEP3 : Inport  Port=2  PortName=EncoderData  Element=Motor3Velocity
  BEP4 : Inport  Port=2  PortName=EncoderData  Element=Motor4Velocity
  Out3 : Outport  PortName=SensorData  Element=Acceleration
  Out1 : Outport  PortName=SensorData  Element=AngularAcceleration
  Out2 : Outport  PortName=SensorData  Element=Pose
  Out4 : Outport  PortName=SensorData  Element=Motor1Velocity
  Out5 : Outport  PortName=SensorData  Element=Motor2Velocity
  Out6 : Outport  PortName=SensorData  Element=Motor3Velocity
  Out7 : Outport  PortName=SensorData  Element=Motor4Velocity
  wires:
  In Bus Element/1 -> Out3/1
  BEP/1 -> Out1/1
  BEP1/1 -> Out2/1
  Bus Element In2/1 -> Out4/1
  BEP2/1 -> Out5/1
  BEP3/1 -> Out6/1
  BEP4/1 -> Out7/1

== system MiniDroneLogicalArchitecture/Minidrone/Main Vehicle/Sensor Module/Encoder ==
  Bus Element In1 : Inport  PortName=PropulsionState
  Bus Element Out1 : Outport  PortName=EncoderData

== system MiniDroneLogicalArchitecture/Minidrone/Main Vehicle/Sensor Module/IMU  ==
  Bus Element Out1 : Outport  PortName=IMUData
